simulink library "IOBlock_Library_TTC580"  (R2021a)
settings: Solver=ode45  StartTime=0.0  StopTime=10.0  RelTol=1e-3
PreLoadFcn:
  | addpath(genpath(fileparts(which('IOBlock_Library_TTC580'))));
  | %addpath(genpath(fileparts(which('IOBlock_Library_TTC580.mdl'))))
  | try
  | addpath(genpath([fileparts(which('IOBlock_Library_TTC580')),'\..\DBC_Importer']));
  | addpath(genpath([fileparts(which('IOBlock_Library_TTC580')),'\..\EEPROM_Importer']));
  | addpath(genpath([fileparts(which('IOBlock_Library_TTC580')),'\..\UserDoc']));
  | catch
  | warning('IOBlock_Library_TTC580: add path to DBC_Importer and EEPROM_Importer manually');
  | end
  | try
  | if exist('..\CustomPackage\scripts\OpenAllPackages.m','file')
  |      run('..\CustomPackage\scripts\OpenAllPackages.m'); %always available, ggf. empty
  | end
  | catch
  | warning('A problem occurred opening automatically the CustomPackage. Please open libraries manually');
  | end
  | try
  | set_param(0,'EditorSmartEditingHotParam','off');
  | catch
  | warning('Simlink preferences for ''Edit key parameter when adding new blocks'' needs to be unchecked manually');
  | end
undefined symbols (not defined in the file or in its folder): ADC_Absolute_10V, ADC_Absolute_32V, ADC_Absolute_5V, ADC_BoardTemp, ADC_ChannelInit, ADC_Current, ADC_Get, ADC_K15_, ADC_Ratiometric_10V, ADC_Ratiometric_5V, ADC_Resistive, ADC_SensorSupply, ADC_UBAT, bit_packing, bit_unpacking, CAN_ConfigMsg, compare2error, compare2FET_PROT_REENABLE, crc32_calc_intern, CRC32_EEPROM_Read, CRC32_EEPROM_Write, DIAG_EnterSafestate, DIAG_Status, DIAG_Status_internal, EEPROM_Mirror, EEPROM_Read, EEPROM_Read_OffsetIn, EEPROM_Read_Raw, EEPROM_Write, EEPROM_Write_OffsetIn, EEPROM_Write_Raw, EnterSafestate, FPU_Handler, Get_DI, Get_DI_VarThreshold, Get_K15_, Get_Pulse_Freq_Curr, Get_Pulse_Freq_Volt, Get_WakeUp, GetDateAndTime, IO_ADC_ResetProtection, IO_Blk_Lib_TTC500, IO_CAN_ReadMsg, IO_CAN_WriteMsg, IO_DI_Get, IO_DI_Init, IO_DI_Init_Var, IO_DO_GetCur, IO_DO_GetVoltage, IO_DO_Init, IO_DO_ResetProtection, IO_DO_Set, IO_Driver_GetSerialNumber, IO_Driver_GetVersionOfDriver, IO_Driver_GetVersionOfFPGA, IO_EEPROM_GetStatus, IO_EEPROM_Init, IO_EEPROM_Read_raw, IO_EEPROM_Write, IO_EEPROM_Write_OffsetIn ... (+73)
libraries: simulink x43
(part 5 of 18)

== system IOBlock_Library_TTC580/System  Blocks TTC580 IOlib ==
  DIAG_Status : Subsystem  LoadFcn=|  mask(DIAG_Status_Code){SampleTime=-1, ttlib=IO_Blk_Lib_TTC500, ttDescription=DIAG_Status, tt_iolib_version=0.16, FPGA_Major=16, FPGA_Minor=5, IODriver_Major=3, IODriver_Minor=1}
      | try
      | %specific upgrade to 0.15
      | if (0.15 > str2num(get_param(gcb,'tt_iolib_version'))) || (0.8 == str2num(get_param(gcb,'tt_iolib_version')))
      |    set_param(gcb,'IODriver_Minor','8'); 
      | end
      | %Upgrade Information - standard BEGIN
      | new_color = 'blue';
      | new_ver = '0.16';
      | act_ver = get_param(gcb,'tt_iolib_version');
      | if not(strcmp(act_ver,new_ver))
      |     disp(['Upgrade block: ',gcb,char(10),'       Version: ',act_ver,' -> ',new_ver]);
      |     %switch - case for specific upgrade information e.g. additional parameter required 
      |     %Change appearance and version information
      |     set_param(gcb,'ForegroundColor',new_color);
      |     set_param(gcb,'tt_iolib_version',new_ver);
      | end
      | %Upgrade Information - standard END
      | catch
      | %Standard catch section BEGIN 
      | disp(' ');
      | disp('------------------------------------------------------------');
      | disp('An error occurred in a callback of the TTC580-BlockLib.');
      | disp(['Please check the parameters in the mask of ',gcb]);
      | disp('If you do not encounter any violations, then please '); 
      | disp('copy the following lines and report this to support@ttcontrol.com ');
      | disp('<< begin of error message dump >>');
      | disp(['Version of TTC580-BlockLib: ', get_param(gcb,'tt_iolib_version')]);
      | disp(get_param(gcb,'ttDescription'));
      | disp(gcb);
      | x=lasterror;disp(x.message);
      | disp(get_param(gcb,'MaskValues'));
      | disp(version);
      | disp(computer);
      | disp('<< end of error message dump >>');
      | disp('------------------------------------------------------------');
      | disp(' ');
      | %Standard catch section END
      | end
      mask help: Status function for diagnostic state machine and watchdog states.
      mask init:
      | %
      settings: CopyFcn=%deleted
      mask Help: web([which('usermanual.html'),'#',lower(get_param(gcb,'ttDescription'))])
      mask Callback FPGA_Major: %
      mask Callback FPGA_Minor: %
      mask Callback IODriver_Major: %
      mask Callback IODriver_Minor: %
  EnterSafestate : Subsystem  mask(EnterSafestate_Code){SampleTime=-1, ttlib=IO_Blk_Lib_TTC500, ttDescription=EnterSafestate, tt_iolib_version=0.8}
      mask help: Allows an application driven safe state.
      mask init:
      | %
      settings: CopyFcn=%deleted
      mask Help: web([which('usermanual.html'),'#',lower(get_param(gcb,'ttDescription'))])
  FPU_Handler : Subsystem  LoadFcn=|  mask(FPU_Handler_Code){SampleTime=-1, ttlib=IO_Blk_Lib_TTC500, ttDescription=FPU_Handler, tt_iolib_version=0.25, division_by_zero=on, input_denormal=off, invalid_operation=on, overflow=on, underflow=off}
      | try
      | %
      | %Upgrade Information - standard BEGIN
      | new_color = 'blue';
      | new_ver = '0.25';
      | act_ver = get_param(gcb,'tt_iolib_version');
      | if not(strcmp(act_ver,new_ver))
      |     disp(['Upgrade block: ',gcb,char(10),'       Version: ',act_ver,' to ',new_ver]);
      |     %switch - case for specific upgrade information e.g. additional parameter required 
      |     %Change appearance and version information
      |     set_param(gcb,'ForegroundColor',new_color);
      |     set_param(gcb,'tt_iolib_version',new_ver);
      | end
      | %Upgrade Information - standard END
      | catch
      | %Standard catch section BEGIN
      | errordlg('An error occurred in a callback of the TTC580-BlockLib. Please open the Diagnostic Viewer for further details');
      | disp(' ');
      | disp('------------------------------------------------------------');
      | disp('An error occurred in a callback of the TTC580-BlockLib.');
      | disp(['Please check the parameters in the mask of ',gcb]);
      | disp('If you do not encounter any violations, then please '); 
      | disp('copy the following lines and report this to support@ttcontrol.com ');
      | disp('<< begin of error message dump >>');
      | disp(['Version of TTC580-BlockLib: ', get_param(gcb,'tt_iolib_version')]);
      | disp(get_param(gcb,'ttDescription'));
      | disp(gcb);
      | x=lasterror;disp(x.message);
      | disp(get_param(gcb,'MaskValues'));
      | disp(version);
      | disp(computer);
      | disp('<< end of error message dump >>');
      | disp('------------------------------------------------------------');
      | disp(' ');
      | %Standard catch section END
      | end
      mask help: Function for FPU exception handler.
      mask init:
      | %
      settings: CopyFcn=%deleted
      mask Help: web([which('usermanual.html'),'#',lower(get_param(gcb,'ttDescription'))])
      mask Callback division_by_zero: %
      mask Callback input_denormal: %
      mask Callback invalid_operation: %
      mask Callback overflow: %
      mask Callback underflow: %
  GetDateAndTime : Subsystem  LoadFcn=|  mask(GetDateAndTime_Code){SampleTime=-1, ttlib=IO_Blk_Lib_TTC500, ttDescription=GetDateAndTime, tt_iolib_version=0.18}
      | try
      | %
      | %Upgrade Information - standard BEGIN
      | new_color = 'blue';
      | new_ver = '0.18';
      | act_ver = get_param(gcb,'tt_iolib_version');
      | if not(strcmp(act_ver,new_ver))
      |     disp(['Upgrade block: ',gcb,char(10),'       Version: ',act_ver,' -> ',new_ver]);
      |     %switch - case for specific upgrade information e.g. additional parameter required 
      |     %Change appearance and version information
      |     set_param(gcb,'ForegroundColor',new_color);
      |     set_param(gcb,'tt_iolib_version',new_ver);
      | end
      | %Upgrade Information - standard END
      | catch
      | %Standard catch section BEGIN 
      | disp(' ');
      | disp('------------------------------------------------------------');
      | disp('An error occurred in a callback of the TTC580-BlockLib.');
      | disp(['Please check the parameters in the mask of ',gcb]);
      | disp('If you do not encounter any violations, then please '); 
      | disp('copy the following lines and report this to support@ttcontrol.com ');
      | disp('<< begin of error message dump >>');
      | disp(['Version of TTC580-BlockLib: ', get_param(gcb,'tt_iolib_version')]);
      | disp(get_param(gcb,'ttDescription'));
      | disp(gcb);
      | x=lasterror;disp(x.message);
      | disp(get_param(gcb,'MaskValues'));
      | disp(version);
      | disp(computer);
      | disp('<< end of error message dump >>');
      | disp('------------------------------------------------------------');
      | disp(' ');
      | %Standard catch section END
      | end
      mask help: Returns the date and time of the real time clock.
      mask init:
      | %
      settings: CopyFcn=%deleted
      mask Help: web([which('usermanual.html'),'#',lower(get_param(gcb,'ttDescription'))])
  IO_Driver_GetSerialNumber : Subsystem  LoadFcn=|  mask(IO_Driver_GetSerialNumber_Code){SampleTime=-1, ttlib=IO_Blk_Lib_TTC500, ttDescription=IO_Driver_GetSerialNumber, tt_iolib_version=0.24}
      | try
      | %
      | %Upgrade Information - standard BEGIN
      | new_color = 'blue';
      | new_ver = '0.24';
      | act_ver = get_param(gcb,'tt_iolib_version');
      | if not(strcmp(act_ver,new_ver))
      |     disp(['Upgrade block: ',gcb,char(10),'       Version: ',act_ver,' -> ',new_ver]);
      |     %switch - case for specific upgrade information e.g. additional parameter required 
      |     %Change appearance and version information
      |     set_param(gcb,'ForegroundColor',new_color);
      |     set_param(gcb,'tt_iolib_version',new_ver);
      | end
      | %Upgrade Information - standard END
      | catch
      | %Standard catch section BEGIN 
      | disp(' ');
      | disp('------------------------------------------------------------');
      | disp('An error occurred in a callback of the TTC580-BlockLib.');
      | disp(['Please check the parameters in the mask of ',gcb]);
      | disp('If you do not encounter any violations, then please '); 
      | disp('copy the following lines and report this to support@ttcontrol.com ');
      | disp('<< begin of error message dump >>');
      | disp(['Version of TTC580-BlockLib: ', get_param(gcb,'tt_iolib_version')]);
      | disp(get_param(gcb,'ttDescription'));
      | disp(gcb);
      | x=lasterror;disp(x.message);
      | disp(get_param(gcb,'MaskValues'));
      | disp(version);
      | disp(computer);
      | disp('<< end of error message dump >>');
      | disp('------------------------------------------------------------');
      | disp(' ');
      | %Standard catch section END
      | end
      mask help: Returns the ECU’s serial number.
      mask init:
      | %
      settings: CopyFcn=%deleted
      mask Help: web([which('usermanual.html'),'#',lower(get_param(gcb,'ttDescription'))])
  MainDlg : Subsystem  LoadFcn=|  mask(MainDlg_CCP_J1939__Code){SampleTime=-1, ttlib=IO_Blk_Lib_TTC500, ttDescription=MainDlg, tt_iolib_version=0.25, baudrate_CAN0=500, tseg1_CAN0=6, tseg2_CAN0=2, sjw_CAN0=1, brp_CAN0=1, baudrate_CAN1=500, tseg1_CAN1=6, tseg2_CAN1=2, sjw_CAN1=1, brp_CAN1=1, baudrate_CAN2=500, tseg1_CAN2=6, tseg2_CAN2=2, sjw_CAN2=1, brp_CAN2=1, baudrate_CAN3=500, baudrate_CAN4=500, baudrate_CAN5=500, baudrate_CAN6=500, tseg1=6, tseg2=2, sjw=1, Duration_ms=10, glitch_filter_time=180, watchdog_window_size=SAFETY_CONF_WINDOW_SIZE_100_PERCENT, watchdog_reset_behavior=SAFETY_CONF_RESETS_DISABLED, brp=0, Enable_sending_DM1_of_J1939=off, DM1_Channel=IO_CAN_CHANNEL_0, J1939SorceAddress=0, DM2_Basis_Address=63488, Show_version_information=off, Major_Number=0, Minor_Number=1, Revison_Number=1, Node_Number=1, Enable_Reset_by_TTCDownloader=on, bFlashOverEthernet=off, Enable_CCP=off, CRO_ID=hex2dec('101'), DTO_ID=hex2dec('102'), CCP_Station_Addr_raw=1, CCP_Station_ID=ECU00001, CPP_channel=IO_CAN_CHANNEL_0, CPP_id_format=IO_CAN_STD_FRAME, bEnable_DAQ0=off, bEnable_DAQ1_2=off, ODT_total=10, bEnable_ErrorCBAction=off, bDIAG_ERR_DISABLE_SSW0=off, bDIAG_ERR_DISABLE_SSW1=off, bDIAG_ERR_DISABLE_SSW2=off}
      | try
      | %
      | %Upgrade Information - standard BEGIN
      | new_color = 'blue';
      | new_ver = '0.25';
      | act_ver = get_param(gcb,'tt_iolib_version');
      | if not(strcmp(act_ver,new_ver))
      |     disp(['Upgrade block: ',gcb,char(10),'       Version: ',act_ver,' to ',new_ver]);
      |     %switch - case for specific upgrade information e.g. additional parameter required 
      |     %Change appearance and version information
      |     set_param(gcb,'ForegroundColor',new_color);
      |     set_param(gcb,'tt_iolib_version',new_ver);
      | end
      | %Upgrade Information - standard END
      | catch
      | %Standard catch section BEGIN
      | errordlg('An error occurred in a callback of the TTC580-BlockLib. Please open the Diagnostic Viewer for further details');
      | disp(' ');
      | disp('------------------------------------------------------------');
      | disp('An error occurred in a callback of the TTC580-BlockLib.');
      | disp(['Please check the parameters in the mask of ',gcb]);
      | disp('If you do not encounter any violations, then please '); 
      | disp('copy the following lines and report this to support@ttcontrol.com ');
      | disp('<< begin of error message dump >>');
      | disp(['Version of TTC580-BlockLib: ', get_param(gcb,'tt_iolib_version')]);
      | disp(get_param(gcb,'ttDescription'));
      | disp(gcb);
      | x=lasterror;disp(x.message);
      | disp(get_param(gcb,'MaskValues'));
      | disp(version);
      | disp(computer);
      | disp('<< end of error message dump >>');
      | disp('------------------------------------------------------------');
      | disp(' ');
      | %Standard catch section END
      | end
      mask prompts: tseg1_CAN0 "tseg1 for CAN0"; tseg2_CAN0 "tseg2 for CAN0"; sjw_CAN0 "sjw for CAN0"; brp_CAN0 "brp for CAN0"; tseg1_CAN1 "tseg1 for CAN1"; tseg2_CAN1 "tseg2 for CAN1"; sjw_CAN1 "sjw for CAN1"; brp_CAN1 "brp for CAN1"; tseg1_CAN2 "tseg1 for CAN2"; tseg2_CAN2 "tseg2 for CAN2"; sjw_CAN2 "sjw for CAN2"; brp_CAN2 "brp for CAN2"; Enable_sending_DM1_of_J1939 "Enable DMx services (J1939)"; DM1_Channel "J1939 channel"; DM2_Basis_Address "Basis Address DM2 [0..63488]"; Show_version_information "Show additional information"; Major_Number "Major Number:"; Minor_Number "Minor Number:"; Revison_Number "Revision Number:"; Node_Number "Node Number:"; Enable_Reset_by_TTCDownloader "Reset by TTC-Downloader"; bFlashOverEthernet "Enable ethernet download requests"; Enable_CCP "Enable CCP"; CRO_ID "CRO ID"; DTO_ID "DTO ID"; CCP_Station_Addr_raw "CCP Station Address"; CCP_Station_ID "CCP Station ID"; CPP_channel "CPP channel"; CPP_id_format "CRO DTO Id format"; bEnable_DAQ0 "Enable DAQ sync"; bEnable_DAQ1_2 "Enable DAQ alternate"; ODT_total "Total ODTs for DAQ lists"; bEnable_ErrorCBAction "Enable dedicated actions for error callback"; bDIAG_ERR_DISABLE_SSW0 "Shut-off group 0"; bDIAG_ERR_DISABLE_SSW1 "Shut-off group 1"; bDIAG_ERR_DISABLE_SSW2 "Shut-off group 2"
      mask help: Block representing main environment-settings of the applications to be run on a TTC580.
      mask init:
      | try
      | %Check if the selected channel is set to 250kBit/s
      | if strcmp(get_param(gcb,'Enable_sending_DM1_of_J1939'),'on')
      |  sChannel = get_param(gcb, 'DM1_Channel');   
      |  cChannelNumber = regexp(sChannel,'(\d)*','match');  %extract numbers
      |  sChannelNumber =  cChannelNumber{end}; %take last number
      |  if ~strcmp(get_param(gcb,['baudrate_CAN',sChannelNumber]),'250')
      |    disp('TTC580-Lib Warning for MainDlg Block: ');
      |    disp(['Setting for baudrate_CAN',sChannelNumber,' is not 250kBit/s as defined in J1939 standard']);
      |    disp('!!!'); 
      | end
      | end
      | if (Duration_ms > 50) || (Duration_ms < 1)
      |     disp('Duration_ms is chosen out of bounds [1..50] !!!');
      | end
      | %swap the Station Address because of Intel format representation due to CCP specification
      | CCP_Station_Addr_raw_loc = str2num(get_param(gcb,'CCP_Station_Addr_raw'));
      | CCP_Station_Addr = swapbytes(uint16(CCP_Station_Addr_raw_loc));%because of big-endian format on the TMS570
      | %%CT>
      | TAG_loc = get_param(gcb,'Tag');
      | if ~isempty(TAG_loc),[~,y]=regexp(TAG_loc,'(^[a-zA-Z0-9_]*)');
      |     if isempty(y) || y~=builtin('length',(TAG_loc)) %don't use length() alone!
      |         error(['The Tag: ',TAG_loc,' needs to start with a letter and may only contain the characters 0-9,a-Z,_ .']);
      | end,end
      | x=find_system(gcbh,'FollowLinks','on','LookUnderMasks','on','BlockType','S-Function');
      | for i=1:builtin('length',(x)) %don't use length() alone!
      |     set_param(x(i),'Tag',TAG_loc);
      | end
      | %<CT%
      | 
      | catch
      | %Standard catch section BEGIN
      | errordlg('An error occurred in a callback of the TTC580-BlockLib. Please open the Diagnostic Viewer for further details');
      | disp(' ');
      | disp('------------------------------------------------------------');
      | disp('An error occurred in a callback of the TTC580-BlockLib.');
      | disp(['Please check the parameters in the mask of ',gcb]);
      | disp('If you do not encounter any violations, then please '); 
      | disp('copy the following lines and report this to support@ttcontrol.com ');
      | disp('<< begin of error message dump >>');
      | disp(['Version of TTC580-BlockLib: ', get_param(gcb,'tt_iolib_version')]);
      | disp(get_param(gcb,'ttDescription'));
      | disp(gcb);
      | x=lasterror;disp(x.message);
      | disp(get_param(gcb,'MaskValues'));
      | disp(version);
      | disp(computer);
      | disp('<< end of error message dump >>');
      | disp('------------------------------------------------------------');
      | disp(' ');
      | %Standard catch section END
      | end
      settings: CopyFcn=%deleted
      mask Help: web([which('usermanual.html'),'#',lower(get_param(gcb,'ttDescription'))])
      mask TypeOptions baudrate_CAN0: 50 | 100 | 125 | 250 | 500 | 1000 | IO_CAN_BIT_USER
      mask Callback baudrate_CAN0:
      | try
      | s_ParameterDecision = 'baudrate_CAN0'; %Deside on this parameter
      | c_ValuesDecision={'50','100','125','250','500','1000'}; %Positive DescitionValues
      | s_ParameterInvisible = {'tseg1_CAN0','tseg2_CAN0','brp_CAN0'}; %Make this invisible
      | %trim
      | if ischar(s_ParameterInvisible)%if secttion for compatibility reasons of template
      |     cs_ParameterInvisible = {s_ParameterInvisible};
      | else
      |     cs_ParameterInvisible = s_ParameterInvisible;
      | end
      | s_ParameterDecision = strtrim(s_ParameterDecision);
      | c_ValuesDecision = strtrim(c_ValuesDecision);
      | for j=1:length(cs_ParameterInvisible)
      |   s_ParameterInvisible = strtrim(cs_ParameterInvisible{j});
      |   c_MaskVisibilities=get_param(gcb,'MaskVisibilities');
      |   %check consistency
      |   idx=strmatch(s_ParameterInvisible,get_param(gcb,'MaskNames'),'exact');
      |   c_MaskVisibilities{idx}='on'; %default
      |     for i = 1: length(c_ValuesDecision)
      |         if ~isempty(strmatch(get_param(gcb, s_ParameterDecision), c_ValuesDecision{i},'exact'))
      |            c_MaskVisibilities{idx}='off';
      |         end
      |     end
      |   set_param(gcb,'MaskVisibilities',c_MaskVisibilities);
      | end
      | catch
      | %Standard catch section BEGIN
      | errordlg('An error occurred in a callback of the TTC580-BlockLib. Please open the Diagnostic Viewer for further details');
      | disp(' ');
      | disp('------------------------------------------------------------');
      | disp('An error occurred in a callback of the TTC580-BlockLib.');
      | disp(['Please check the parameters in the mask of ',gcb]);
      | disp('If you do not encounter any violations, then please ');
      | disp('copy the following lines and report this to support@ttcontrol.com ');
      | disp('<< begin of error message dump >>');
      | disp(['Version of TTC580-BlockLib: ', get_param(gcb,'tt_iolib_version')]);
      | disp(get_param(gcb,'ttDescription'));
      | disp(gcb);
      | x=lasterror;disp(x.message);
      | disp(get_param(gcb,'MaskValues'));
      | disp(version);
      | disp(computer);
      | disp('<< end of error message dump >>');
      | disp('------------------------------------------------------------');
      | disp(' ');
      | %Standard catch section END
      | end
      mask TypeOptions tseg1_CAN0: 3 | 4 | 5 | 6 | 7 | 8 | 9 | 10 | 11 | 12 | 13 | 14 | 15 | 16
      mask Callback tseg1_CAN0: %
      mask TypeOptions tseg2_CAN0: 2 | 3 | 4 | 5 | 6 | 7 | 8
      mask Callback tseg2_CAN0: %
      mask TypeOptions sjw_CAN0: 1 | 2 | 3 | 4
      mask Callback sjw_CAN0: %
      mask TypeOptions brp_CAN0: 1 | 2 | 3 | 4 | 5 | 6 | 7 | 8 | 9 | 10 | 11 | 12 | 13 | 14 | 15 | 16 | 17 | 18 | 19 | 20 | 21 | 22 | 23 | 24 | 25 | 26 | 27 | 28 | 29 | 30 | 31 | 32 | 33 | 34 | 35 | 36 | 37 | 38 | 39 | 40 | 41 | 42 | 43 | 44 | 45 | 46 | 47 | 48 | 49 | 50 | 51 | 52 | 53 | 54 | 55 | 56 | 57 | 58 | 59 | 60 | 61 | 62 | 63 | 64
      mask Callback brp_CAN0: %
      mask TypeOptions baudrate_CAN1: 50 | 100 | 125 | 250 | 500 | 1000 | IO_CAN_BIT_USER
      mask Callback baudrate_CAN1:
      | try
      | s_ParameterDecision = 'baudrate_CAN1'; %Deside on this parameter
      | c_ValuesDecision={'50','100','125','250','500','1000'}; %Positive DescitionValues
      | s_ParameterInvisible = {'tseg1_CAN1','tseg2_CAN1','brp_CAN1'}; %Make this invisible
      | %trim
      | if ischar(s_ParameterInvisible)%if secttion for compatibility reasons of template
      |     cs_ParameterInvisible = {s_ParameterInvisible};
      | else
      |     cs_ParameterInvisible = s_ParameterInvisible;
      | end
      | s_ParameterDecision = strtrim(s_ParameterDecision);
      | c_ValuesDecision = strtrim(c_ValuesDecision);
      | for j=1:length(cs_ParameterInvisible)
      |   s_ParameterInvisible = strtrim(cs_ParameterInvisible{j});
      |   c_MaskVisibilities=get_param(gcb,'MaskVisibilities');
      |   %check consistency
      |   idx=strmatch(s_ParameterInvisible,get_param(gcb,'MaskNames'),'exact');
      |   c_MaskVisibilities{idx}='on'; %default
      |     for i = 1: length(c_ValuesDecision)
      |         if ~isempty(strmatch(get_param(gcb, s_ParameterDecision), c_ValuesDecision{i},'exact'))
      |            c_MaskVisibilities{idx}='off';
      |         end
      |     end
      |   set_param(gcb,'MaskVisibilities',c_MaskVisibilities);
      | end
      | catch
      | %Standard catch section BEGIN
      | errordlg('An error occurred in a callback of the TTC580-BlockLib. Please open the Diagnostic Viewer for further details');
      | disp(' ');
      | disp('------------------------------------------------------------');
      | disp('An error occurred in a callback of the TTC580-BlockLib.');
      | disp(['Please check the parameters in the mask of ',gcb]);
      | disp('If you do not encounter any violations, then please ');
      | disp('copy the following lines and report this to support@ttcontrol.com ');
      | disp('<< begin of error message dump >>');
      | disp(['Version of TTC580-BlockLib: ', get_param(gcb,'tt_iolib_version')]);
      | disp(get_param(gcb,'ttDescription'));
      | disp(gcb);
      | x=lasterror;disp(x.message);
      | disp(get_param(gcb,'MaskValues'));
      | disp(version);
      | disp(computer);
      | disp('<< end of error message dump >>');
      | disp('------------------------------------------------------------');
      | disp(' ');
      | %Standard catch section END
      | end
      mask TypeOptions tseg1_CAN1: 3 | 4 | 5 | 6 | 7 | 8 | 9 | 10 | 11 | 12 | 13 | 14 | 15 | 16
      mask Callback tseg1_CAN1: %
      mask TypeOptions tseg2_CAN1: 2 | 3 | 4 | 5 | 6 | 7 | 8
      mask Callback tseg2_CAN1: %
      mask TypeOptions sjw_CAN1: 1 | 2 | 3 | 4
      mask Callback sjw_CAN1: %
      mask TypeOptions brp_CAN1: 1 | 2 | 3 | 4 | 5 | 6 | 7 | 8 | 9 | 10 | 11 | 12 | 13 | 14 | 15 | 16 | 17 | 18 | 19 | 20 | 21 | 22 | 23 | 24 | 25 | 26 | 27 | 28 | 29 | 30 | 31 | 32 | 33 | 34 | 35 | 36 | 37 | 38 | 39 | 40 | 41 | 42 | 43 | 44 | 45 | 46 | 47 | 48 | 49 | 50 | 51 | 52 | 53 | 54 | 55 | 56 | 57 | 58 | 59 | 60 | 61 | 62 | 63 | 64
      mask Callback brp_CAN1: %
      mask TypeOptions baudrate_CAN2: 50 | 100 | 125 | 250 | 500 | 1000 | IO_CAN_BIT_USER
      mask Callback baudrate_CAN2:
      | try
      | s_ParameterDecision = 'baudrate_CAN2'; %Deside on this parameter
      | c_ValuesDecision={'50','100','125','250','500','1000'}; %Positive DescitionValues
      | s_ParameterInvisible = {'tseg1_CAN2','tseg2_CAN2','brp_CAN2'}; %Make this invisible
      | %trim
      | if ischar(s_ParameterInvisible)%if secttion for compatibility reasons of template
      |     cs_ParameterInvisible = {s_ParameterInvisible};
      | else
      |     cs_ParameterInvisible = s_ParameterInvisible;
      | end
      | s_ParameterDecision = strtrim(s_ParameterDecision);
      | c_ValuesDecision = strtrim(c_ValuesDecision);
      | for j=1:length(cs_ParameterInvisible)
      |   s_ParameterInvisible = strtrim(cs_ParameterInvisible{j});
      |   c_MaskVisibilities=get_param(gcb,'MaskVisibilities');
      |   %check consistency
      |   idx=strmatch(s_ParameterInvisible,get_param(gcb,'MaskNames'),'exact');
      |   c_MaskVisibilities{idx}='on'; %default
      |     for i = 1: length(c_ValuesDecision)
      |         if ~isempty(strmatch(get_param(gcb, s_ParameterDecision), c_ValuesDecision{i},'exact'))
      |            c_MaskVisibilities{idx}='off';
      |         end
      |     end
      |   set_param(gcb,'MaskVisibilities',c_MaskVisibilities);
      | end
      | catch
      | %Standard catch section BEGIN
      | errordlg('An error occurred in a callback of the TTC580-BlockLib. Please open the Diagnostic Viewer for further details');
      | disp(' ');
      | disp('------------------------------------------------------------');
      | disp('An error occurred in a callback of the TTC580-BlockLib.');
      | disp(['Please check the parameters in the mask of ',gcb]);
      | disp('If you do not encounter any violations, then please ');
      | disp('copy the following lines and report this to support@ttcontrol.com ');
      | disp('<< begin of error message dump >>');
      | disp(['Version of TTC580-BlockLib: ', get_param(gcb,'tt_iolib_version')]);
      | disp(get_param(gcb,'ttDescription'));
      | disp(gcb);
      | x=lasterror;disp(x.message);
      | disp(get_param(gcb,'MaskValues'));
      | disp(version);
      | disp(computer);
      | disp('<< end of error message dump >>');
      | disp('------------------------------------------------------------');
      | disp(' ');
      | %Standard catch section END
      | end
      mask TypeOptions tseg1_CAN2: 3 | 4 | 5 | 6 | 7 | 8 | 9 | 10 | 11 | 12 | 13 | 14 | 15 | 16
      mask Callback tseg1_CAN2: %
      mask TypeOptions tseg2_CAN2: 2 | 3 | 4 | 5 | 6 | 7 | 8
      mask Callback tseg2_CAN2: %
      mask TypeOptions sjw_CAN2: 1 | 2 | 3 | 4
      mask Callback sjw_CAN2: %
      mask TypeOptions brp_CAN2: 1 | 2 | 3 | 4 | 5 | 6 | 7 | 8 | 9 | 10 | 11 | 12 | 13 | 14 | 15 | 16 | 17 | 18 | 19 | 20 | 21 | 22 | 23 | 24 | 25 | 26 | 27 | 28 | 29 | 30 | 31 | 32 | 33 | 34 | 35 | 36 | 37 | 38 | 39 | 40 | 41 | 42 | 43 | 44 | 45 | 46 | 47 | 48 | 49 | 50 | 51 | 52 | 53 | 54 | 55 | 56 | 57 | 58 | 59 | 60 | 61 | 62 | 63 | 64
      mask Callback brp_CAN2: %
      mask TypeOptions baudrate_CAN3: 50 | 100 | 125 | 250 | 500 | 1000
      mask Callback baudrate_CAN3: %
      mask TypeOptions baudrate_CAN4: 50 | 100 | 125 | 250 | 500 | 1000
      mask Callback baudrate_CAN4: %
      mask TypeOptions baudrate_CAN5: 50 | 100 | 125 | 250 | 500 | 1000
      mask Callback baudrate_CAN5: %
      mask TypeOptions baudrate_CAN6: 50 | 100 | 125 | 250 | 500 | 1000
      mask Callback baudrate_CAN6: %
      mask TypeOptions tseg1: 3 | 4 | 5 | 6 | 7 | 8 | 9 | 10 | 11 | 12 | 13 | 14 | 15 | 16
      mask Callback tseg1: %
      mask TypeOptions tseg2: 2 | 3 | 4 | 5 | 6 | 7 | 8
      mask Callback tseg2: %
      mask TypeOptions sjw: 1 | 2 | 3 | 4
      mask Callback sjw: %
      mask Callback Duration_ms: %
      mask Callback glitch_filter_time: %
      mask TypeOptions watchdog_window_size: SAFETY_CONF_WINDOW_SIZE_100_PERCENT | SAFETY_CONF_WINDOW_SIZE_50_PERCENT | SAFETY_CONF_WINDOW_SIZE_25_PERCENT | SAFETY_CONF_WINDOW_SIZE_12_5_PERCENT | SAFETY_CONF_WINDOW_SIZE_6_25_PERCENT | SAFETY_CONF_WINDOW_SIZE_3_125_PERCENT
      mask Callback watchdog_window_size: %
      mask Callback watchdog_reset_behavior: %
      mask Callback brp: %
      mask Callback Enable_sending_DM1_of_J1939:
      | try
      | s_ParameterDecision = 'Enable_sending_DM1_of_J1939'; %Deside on this parameter
      | c_ValuesDecision={'off'}; %Positive DescitionValues
      | s_ParameterInvisible = 'DM1_Channel'; %Make this invisible
      | %trim
      | if ischar(s_ParameterInvisible)%if secttion for compatibility reasons of template
      |     cs_ParameterInvisible = {s_ParameterInvisible};
      | else
      |     cs_ParameterInvisible = s_ParameterInvisible;
      | end
      | s_ParameterDecision = strtrim(s_ParameterDecision);
      | c_ValuesDecision = strtrim(c_ValuesDecision);
      | for j=1:length(cs_ParameterInvisible)
      |   s_ParameterInvisible = strtrim(cs_ParameterInvisible{j});
      |   c_MaskVisibilities=get_param(gcb,'MaskVisibilities');
      |   %check consistency
      |   idx=strmatch(s_ParameterInvisible,get_param(gcb,'MaskNames'),'exact');
      |   c_MaskVisibilities{idx}='on'; %default
      |     for i = 1: length(c_ValuesDecision)
      |         if ~isempty(strmatch(get_param(gcb, s_ParameterDecision), c_ValuesDecision{i},'exact'))
      |            c_MaskVisibilities{idx}='off';
      |         end
      |     end
      |   set_param(gcb,'MaskVisibilities',c_MaskVisibilities);
      | end
      | s_ParameterDecision = 'Enable_sending_DM1_of_J1939'; %Deside on this parameter
      | c_ValuesDecision={'off'}; %Positive DescitionValues
      | s_ParameterInvisible = 'J1939SorceAddress'; %Make this invisible
      | %trim
      | if ischar(s_ParameterInvisible)%if secttion for compatibility reasons of template
      |     cs_ParameterInvisible = {s_ParameterInvisible};
      | else
      |     cs_ParameterInvisible = s_ParameterInvisible;
      | end
      | s_ParameterDecision = strtrim(s_ParameterDecision);
      | c_ValuesDecision = strtrim(c_ValuesDecision);
      | for j=1:length(cs_ParameterInvisible)
      |   s_ParameterInvisible = strtrim(cs_ParameterInvisible{j});
      |   c_MaskVisibilities=get_param(gcb,'MaskVisibilities');
      |   %check consistency
      |   idx=strmatch(s_ParameterInvisible,get_param(gcb,'MaskNames'),'exact');
      |   c_MaskVisibilities{idx}='on'; %default
      |     for i = 1: length(c_ValuesDecision)
      |         if ~isempty(strmatch(get_param(gcb, s_ParameterDecision), c_ValuesDecision{i},'exact'))
      |            c_MaskVisibilities{idx}='off';
      |         end
      |     end
      |   set_param(gcb,'MaskVisibilities',c_MaskVisibilities);
      | end
      | s_ParameterDecision = 'Enable_sending_DM1_of_J1939'; %Deside on this parameter
      | c_ValuesDecision={'off'}; %Positive DescitionValues
      | s_ParameterInvisible = 'DM2_Basis_Address'; %Make this invisible
      | %trim
      | if ischar(s_ParameterInvisible)%if secttion for compatibility reasons of template
      |     cs_ParameterInvisible = {s_ParameterInvisible};
      | else
      |     cs_ParameterInvisible = s_ParameterInvisible;
      | end
      | s_ParameterDecision = strtrim(s_ParameterDecision);
      | c_ValuesDecision = strtrim(c_ValuesDecision);
      | for j=1:length(cs_ParameterInvisible)
      |   s_ParameterInvisible = strtrim(cs_ParameterInvisible{j});
      |   c_MaskVisibilities=get_param(gcb,'MaskVisibilities');
      |   %check consistency
      |   idx=strmatch(s_ParameterInvisible,get_param(gcb,'MaskNames'),'exact');
      |   c_MaskVisibilities{idx}='on'; %default
      |     for i = 1: length(c_ValuesDecision)
      |         if ~isempty(strmatch(get_param(gcb, s_ParameterDecision), c_ValuesDecision{i},'exact'))
      |            c_MaskVisibilities{idx}='off';
      |         end
      |     end
      |   set_param(gcb,'MaskVisibilities',c_MaskVisibilities);
      | end
      | catch
      | %Standard catch section BEGIN
      | errordlg('An error occurred in a callback of the TTC580-BlockLib. Please open the Diagnostic Viewer for further details');
      | disp(' ');
      | disp('------------------------------------------------------------');
      | disp('An error occurred in a callback of the TTC580-BlockLib.');
      | disp(['Please check the parameters in the mask of ',gcb]);
      | disp('If you do not encounter any violations, then please ');
      | disp('copy the following lines and report this to support@ttcontrol.com ');
      | disp('<< begin of error message dump >>');
      | disp(['Version of TTC580-BlockLib: ', get_param(gcb,'tt_iolib_version')]);
      | disp(get_param(gcb,'ttDescription'));
      | disp(gcb);
      | x=lasterror;disp(x.message);
      | disp(get_param(gcb,'MaskValues'));
      | disp(version);
      | disp(computer);
      | disp('<< end of error message dump >>');
      | disp('------------------------------------------------------------');
      | disp(' ');
      | %Standard catch section END
      | end
      mask TypeOptions DM1_Channel: IO_CAN_CHANNEL_0  | IO_CAN_CHANNEL_1 | IO_CAN_CHANNEL_2 | IO_CAN_CHANNEL_3 | IO_CAN_CHANNEL_4 | IO_CAN_CHANNEL_5 | IO_CAN_CHANNEL_6
      mask Callback DM1_Channel: %
      mask Callback J1939SorceAddress: %
      mask Callback DM2_Basis_Address:
      | try
      | sParam = 'DM2_Basis_Address';
      | vBounds = [0,63488];
      | iValue = str2num(get_param(gcb,sParam));
      | if (iValue > vBounds(2))
      |     disp(['Value of ',sParam,' is chosen out of bounds [',num2str(vBounds(1)),'..',num2str(vBounds(2)),'] -> set to maximum possible !!!']);
      |     iValue = vBounds(2); %set to maximum
      |     set_param(gcb,sParam,num2str(iValue));
      | elseif (iValue < vBounds(1))
      |     disp(['Value of ',sParam,' is chosen out of bounds [',num2str(vBounds(1)),'..',num2str(vBounds(2)),'] -> set to minimum possible !!!']);
      |     iValue = vBounds(1); %set to minimum
      |     set_param(gcb,sParam,num2str(iValue));
      | end
      | catch
      | %Standard catch section BEGIN
      | errordlg('An error occurred in a callback of the TTC580-BlockLib. Please open the Diagnostic Viewer for further details');
      | disp(' ');
      | disp('------------------------------------------------------------');
      | disp('An error occurred in a callback of the TTC580-BlockLib.');
      | disp(['Please check the parameters in the mask of ',gcb]);
      | disp('If you do not encounter any violations, then please ');
      | disp('copy the following lines and report this to support@ttcontrol.com ');
      | disp('<< begin of error message dump >>');
      | disp(['Version of TTC580-BlockLib: ', get_param(gcb,'tt_iolib_version')]);
      | disp(get_param(gcb,'ttDescription'));
      | disp(gcb);
      | x=lasterror;disp(x.message);
      | disp(get_param(gcb,'MaskValues'));
      | disp(version);
      | disp(computer);
      | disp('<< end of error message dump >>');
      | disp('------------------------------------------------------------');
      | disp(' ');
      | %Standard catch section END
      | end
      mask Callback Show_version_information:
      | try
      | s_ParameterDecision = 'Show_version_information'; %Deside on this parameter
      | c_ValuesDecision={'off'}; %Positive DescitionValues
      | s_ParameterInvisible = 'Major_Number'; %Make this invisible
      | %trim
      | if ischar(s_ParameterInvisible)%if secttion for compatibility reasons of template
      |     cs_ParameterInvisible = {s_ParameterInvisible};
      | else
      |     cs_ParameterInvisible = s_ParameterInvisible;
      | end
      | s_ParameterDecision = strtrim(s_ParameterDecision);
      | c_ValuesDecision = strtrim(c_ValuesDecision);
      | for j=1:length(cs_ParameterInvisible)
      |   s_ParameterInvisible = strtrim(cs_ParameterInvisible{j});
      |   c_MaskVisibilities=get_param(gcb,'MaskVisibilities');
      |   %check consistency
      |   idx=strmatch(s_ParameterInvisible,get_param(gcb,'MaskNames'),'exact');
      |   c_MaskVisibilities{idx}='on'; %default
      |     for i = 1: length(c_ValuesDecision)
      |         if ~isempty(strmatch(get_param(gcb, s_ParameterDecision), c_ValuesDecision{i},'exact'))
      |            c_MaskVisibilities{idx}='off';
      |         end
      |     end
      |   set_param(gcb,'MaskVisibilities',c_MaskVisibilities);
      | end
      | s_ParameterDecision = 'Show_version_information'; %Deside on this parameter
      | c_ValuesDecision={'off'}; %Positive DescitionValues
      | s_ParameterInvisible = 'Minor_Number'; %Make this invisible
      | %trim
      | if ischar(s_ParameterInvisible)%if secttion for compatibility reasons of template
      |     cs_ParameterInvisible = {s_ParameterInvisible};
      | else
      |     cs_ParameterInvisible = s_ParameterInvisible;
      | end
      | s_ParameterDecision = strtrim(s_ParameterDecision);
      | c_ValuesDecision = strtrim(c_ValuesDecision);
      | for j=1:length(cs_ParameterInvisible)
      |   s_ParameterInvisible = strtrim(cs_ParameterInvisible{j});
      |   c_MaskVisibilities=get_param(gcb,'MaskVisibilities');
      |   %check consistency
      |   idx=strmatch(s_ParameterInvisible,get_param(gcb,'MaskNames'),'exact');
      |   c_MaskVisibilities{idx}='on'; %default
      |     for i = 1: length(c_ValuesDecision)
      |         if ~isempty(strmatch(get_param(gcb, s_ParameterDecision), c_ValuesDecision{i},'exact'))
      |            c_MaskVisibilities{idx}='off';
      |         end
      |     end
      |   set_param(gcb,'MaskVisibilities',c_MaskVisibilities);
      | end
      | s_ParameterDecision = 'Show_version_information'; %Deside on this parameter
      | c_ValuesDecision={'off'}; %Positive DescitionValues
      | s_ParameterInvisible = 'Revison_Number'; %Make this invisible
      | %trim
      | if ischar(s_ParameterInvisible)%if secttion for compatibility reasons of template
      |     cs_ParameterInvisible = {s_ParameterInvisible};
      | else
      |     cs_ParameterInvisible = s_ParameterInvisible;
      | end
      | s_ParameterDecision = strtrim(s_ParameterDecision);
      | c_ValuesDecision = strtrim(c_ValuesDecision);
      | for j=1:length(cs_ParameterInvisible)
      |   s_ParameterInvisible = strtrim(cs_ParameterInvisible{j});
      |   c_MaskVisibilities=get_param(gcb,'MaskVisibilities');
      |   %check consistency
      |   idx=strmatch(s_ParameterInvisible,get_param(gcb,'MaskNames'),'exact');
      |   c_MaskVisibilities{idx}='on'; %default
      |     for i = 1: length(c_ValuesDecision)
      |         if ~isempty(strmatch(get_param(gcb, s_ParameterDecision), c_ValuesDecision{i},'exact'))
      |            c_MaskVisibilities{idx}='off';
      |         end
      |     end
      |   set_param(gcb,'MaskVisibilities',c_MaskVisibilities);
      | end
      | s_ParameterDecision = 'Show_version_information'; %Deside on this parameter
      | c_ValuesDecision={'off'}; %Positive DescitionValues
      | s_ParameterInvisible = 'Node_Number'; %Make this invisible
      | %trim
      | if ischar(s_ParameterInvisible)%if secttion for compatibility reasons of template
      |     cs_ParameterInvisible = {s_ParameterInvisible};
      | else
      |     cs_ParameterInvisible = s_ParameterInvisible;
      | end
      | s_ParameterDecision = strtrim(s_ParameterDecision);
      | c_ValuesDecision = strtrim(c_ValuesDecision);
      | for j=1:length(cs_ParameterInvisible)
      |   s_ParameterInvisible = strtrim(cs_ParameterInvisible{j});
      |   c_MaskVisibilities=get_param(gcb,'MaskVisibilities');
      |   %check consistency
      |   idx=strmatch(s_ParameterInvisible,get_param(gcb,'MaskNames'),'exact');
      |   c_MaskVisibilities{idx}='on'; %default
      |     for i = 1: length(c_ValuesDecision)
      |         if ~isempty(strmatch(get_param(gcb, s_ParameterDecision), c_ValuesDecision{i},'exact'))
      |            c_MaskVisibilities{idx}='off';
      |         end
      |     end
      |   set_param(gcb,'MaskVisibilities',c_MaskVisibilities);
      | end
      | catch
      | %Standard catch section BEGIN
      | errordlg('An error occurred in a callback of the TTC580-BlockLib. Please open the Diagnostic Viewer for further details');
      | disp(' ');
      | disp('------------------------------------------------------------');
      | disp('An error occurred in a callback of the TTC580-BlockLib.');
      | disp(['Please check the parameters in the mask of ',gcb]);
      | disp('If you do not encounter any violations, then please ');
      | disp('copy the following lines and report this to support@ttcontrol.com ');
      | disp('<< begin of error message dump >>');
      | disp(['Version of TTC580-BlockLib: ', get_param(gcb,'tt_iolib_version')]);
      | disp(get_param(gcb,'ttDescription'));
      | disp(gcb);
      | x=lasterror;disp(x.message);
      | disp(get_param(gcb,'MaskValues'));
      | disp(version);
      | disp(computer);
      | disp('<< end of error message dump >>');
      | disp('------------------------------------------------------------');
      | disp(' ');
      | %Standard catch section END
      | end
      mask Callback Major_Number: %
      mask Callback Minor_Number: %
      mask Callback Revison_Number: %
      mask Callback Node_Number: %
      mask Callback Enable_Reset_by_TTCDownloader:
      | try
      | s_ParameterDecision = 'Enable_Reset_by_TTCDownloader'; %Deside on this parameter
      | c_ValuesDecision={'on'}; %Positive DescitionValues
      | s_ParameterInvisible = 'bFlashOverEthernet'; %Make this invisible
      | %trim
      | if ischar(s_ParameterInvisible)%if secttion for compatibility reasons of template
      |     cs_ParameterInvisible = {s_ParameterInvisible};
      | else
      |     cs_ParameterInvisible = s_ParameterInvisible;
      | end
      | s_ParameterDecision = strtrim(s_ParameterDecision);
      | c_ValuesDecision = strtrim(c_ValuesDecision);
      | for j=1:length(cs_ParameterInvisible)
      |   s_ParameterInvisible = strtrim(cs_ParameterInvisible{j});
      |   c_MaskVisibilities=get_param(gcb,'MaskVisibilities');
      |   %check consistency
      |   idx=strmatch(s_ParameterInvisible,get_param(gcb,'MaskNames'),'exact');
      |   c_MaskVisibilities{idx}='on'; %default
      |     for i = 1: length(c_ValuesDecision)
      |         if ~isempty(strmatch(get_param(gcb, s_ParameterDecision), c_ValuesDecision{i},'exact'))
      |            c_MaskVisibilities{idx}='off';
      |         end
      |     end
      |   set_param(gcb,'MaskVisibilities',c_MaskVisibilities);
      | end
      | catch
      | %Standard catch section BEGIN
      | errordlg('An error occurred in a callback of the TTC580-BlockLib. Please open the Diagnostic Viewer for further details');
      | disp(' ');
      | disp('------------------------------------------------------------');
      | disp('An error occurred in a callback of the TTC580-BlockLib.');
      | disp(['Please check the parameters in the mask of ',gcb]);
      | disp('If you do not encounter any violations, then please ');
      | disp('copy the following lines and report this to support@ttcontrol.com ');
      | disp('<< begin of error message dump >>');
      | disp(['Version of TTC580-BlockLib: ', get_param(gcb,'tt_iolib_version')]);
      | disp(get_param(gcb,'ttDescription'));
      | disp(gcb);
      | x=lasterror;disp(x.message);
      | disp(get_param(gcb,'MaskValues'));
      | disp(version);
      | disp(computer);
      | disp('<< end of error message dump >>');
      | disp('------------------------------------------------------------');
      | disp(' ');
      | %Standard catch section END
      | end
      mask Callback bFlashOverEthernet:
      | try
      | s_ParameterDecision = 'bFlashOverEthernet'; %Deside on this parameter
      | c_ValuesDecision={'on'}; %Positive DescitionValues
      | s_ParameterInvisible = 'Enable_Reset_by_TTCDownloader'; %Make this invisible
      | %trim
      | if ischar(s_ParameterInvisible)%if secttion for compatibility reasons of template
      |     cs_ParameterInvisible = {s_ParameterInvisible};
      | else
      |     cs_ParameterInvisible = s_ParameterInvisible;
      | end
      | s_ParameterDecision = strtrim(s_ParameterDecision);
      | c_ValuesDecision = strtrim(c_ValuesDecision);
      | for j=1:length(cs_ParameterInvisible)
      |   s_ParameterInvisible = strtrim(cs_ParameterInvisible{j});
      |   c_MaskVisibilities=get_param(gcb,'MaskVisibilities');
      |   %check consistency
      |   idx=strmatch(s_ParameterInvisible,get_param(gcb,'MaskNames'),'exact');
      |   c_MaskVisibilities{idx}='on'; %default
      |     for i = 1: length(c_ValuesDecision)
      |         if ~isempty(strmatch(get_param(gcb, s_ParameterDecision), c_ValuesDecision{i},'exact'))
      |            c_MaskVisibilities{idx}='off';
      |         end
      |     end
      |   set_param(gcb,'MaskVisibilities',c_MaskVisibilities);
      | end
      | catch
      | %Standard catch section BEGIN
      | errordlg('An error occurred in a callback of the TTC580-BlockLib. Please open the Diagnostic Viewer for further details');
      | disp(' ');
      | disp('------------------------------------------------------------');
      | disp('An error occurred in a callback of the TTC580-BlockLib.');
      | disp(['Please check the parameters in the mask of ',gcb]);
      | disp('If you do not encounter any violations, then please ');
      | disp('copy the following lines and report this to support@ttcontrol.com ');
      | disp('<< begin of error message dump >>');
      | disp(['Version of TTC580-BlockLib: ', get_param(gcb,'tt_iolib_version')]);
      | disp(get_param(gcb,'ttDescription'));
      | disp(gcb);
      | x=lasterror;disp(x.message);
      | disp(get_param(gcb,'MaskValues'));
      | disp(version);
      | disp(computer);
      | disp('<< end of error message dump >>');
      | disp('------------------------------------------------------------');
      | disp(' ');
      | %Standard catch section END
      | end
      mask Callback Enable_CCP:
      | try
      | s_ParameterDecision = 'Enable_CCP'; %Deside on this parameter
      | c_ValuesDecision={'off'}; %Positive DescitionValues
      | s_ParameterInvisible = 'CRO_ID'; %Make this invisible
      | %trim
      | if ischar(s_ParameterInvisible)%if secttion for compatibility reasons of template
      |     cs_ParameterInvisible = {s_ParameterInvisible};
      | else
      |     cs_ParameterInvisible = s_ParameterInvisible;
      | end
      | s_ParameterDecision = strtrim(s_ParameterDecision);
      | c_ValuesDecision = strtrim(c_ValuesDecision);
      | for j=1:length(cs_ParameterInvisible)
      |   s_ParameterInvisible = strtrim(cs_ParameterInvisible{j});
      |   c_MaskVisibilities=get_param(gcb,'MaskVisibilities');
      |   %check consistency
      |   idx=strmatch(s_ParameterInvisible,get_param(gcb,'MaskNames'),'exact');
      |   c_MaskVisibilities{idx}='on'; %default
      |     for i = 1: length(c_ValuesDecision)
      |         if ~isempty(strmatch(get_param(gcb, s_ParameterDecision), c_ValuesDecision{i},'exact'))
      |            c_MaskVisibilities{idx}='off';
      |         end
      |     end
      |   set_param(gcb,'MaskVisibilities',c_MaskVisibilities);
      | end
      | s_ParameterDecision = 'Enable_CCP'; %Deside on this parameter
      | c_ValuesDecision={'off'}; %Positive DescitionValues
      | s_ParameterInvisible = 'DTO_ID'; %Make this invisible
      | %trim
      | if ischar(s_ParameterInvisible)%if secttion for compatibility reasons of template
      |     cs_ParameterInvisible = {s_ParameterInvisible};
      | else
      |     cs_ParameterInvisible = s_ParameterInvisible;
      | end
      | s_ParameterDecision = strtrim(s_ParameterDecision);
      | c_ValuesDecision = strtrim(c_ValuesDecision);
      | for j=1:length(cs_ParameterInvisible)
      |   s_ParameterInvisible = strtrim(cs_ParameterInvisible{j});
      |   c_MaskVisibilities=get_param(gcb,'MaskVisibilities');
      |   %check consistency
      |   idx=strmatch(s_ParameterInvisible,get_param(gcb,'MaskNames'),'exact');
      |   c_MaskVisibilities{idx}='on'; %default
      |     for i = 1: length(c_ValuesDecision)
      |         if ~isempty(strmatch(get_param(gcb, s_ParameterDecision), c_ValuesDecision{i},'exact'))
      |            c_MaskVisibilities{idx}='off';
      |         end
      |     end
      |   set_param(gcb,'MaskVisibilities',c_MaskVisibilities);
      | end
      | s_ParameterDecision = 'Enable_CCP'; %Deside on this parameter
      | c_ValuesDecision={'off'}; %Positive DescitionValues
      | s_ParameterInvisible = 'CCP_Station_Addr_raw'; %Make this invisible
      | %trim
      | if ischar(s_ParameterInvisible)%if secttion for compatibility reasons of template
      |     cs_ParameterInvisible = {s_ParameterInvisible};
      | else
      |     cs_ParameterInvisible = s_ParameterInvisible;
      | end
      | s_ParameterDecision = strtrim(s_ParameterDecision);
      | c_ValuesDecision = strtrim(c_ValuesDecision);
      | for j=1:length(cs_ParameterInvisible)
      |   s_ParameterInvisible = strtrim(cs_ParameterInvisible{j});
      |   c_MaskVisibilities=get_param(gcb,'MaskVisibilities');
      |   %check consistency
      |   idx=strmatch(s_ParameterInvisible,get_param(gcb,'MaskNames'),'exact');
      |   c_MaskVisibilities{idx}='on'; %default
      |     for i = 1: length(c_ValuesDecision)
      |         if ~isempty(strmatch(get_param(gcb, s_ParameterDecision), c_ValuesDecision{i},'exact'))
      |            c_MaskVisibilities{idx}='off';
      |         end
      |     end
      |   set_param(gcb,'MaskVisibilities',c_MaskVisibilities);
      | end
      | s_ParameterDecision = 'Enable_CCP'; %Deside on this parameter
      | c_ValuesDecision={'off'}; %Positive DescitionValues
      | s_ParameterInvisible = 'CCP_Station_ID'; %Make this invisible
      | %trim
      | if ischar(s_ParameterInvisible)%if secttion for compatibility reasons of template
      |     cs_ParameterInvisible = {s_ParameterInvisible};
      | else
      |     cs_ParameterInvisible = s_ParameterInvisible;
      | end
      | s_ParameterDecision = strtrim(s_ParameterDecision);
      | c_ValuesDecision = strtrim(c_ValuesDecision);
      | for j=1:length(cs_ParameterInvisible)
      |   s_ParameterInvisible = strtrim(cs_ParameterInvisible{j});
      |   c_MaskVisibilities=get_param(gcb,'MaskVisibilities');
      |   %check consistency
      |   idx=strmatch(s_ParameterInvisible,get_param(gcb,'MaskNames'),'exact');
      |   c_MaskVisibilities{idx}='on'; %default
      |     for i = 1: length(c_ValuesDecision)
      |         if ~isempty(strmatch(get_param(gcb, s_ParameterDecision), c_ValuesDecision{i},'exact'))
      |            c_MaskVisibilities{idx}='off';
      |         end
      |     end
      |   set_param(gcb,'MaskVisibilities',c_MaskVisibilities);
      | end
      | s_ParameterDecision = 'Enable_CCP'; %Deside on this parameter
      | c_ValuesDecision={'off'}; %Positive DescitionValues
      | s_ParameterInvisible = 'CPP_channel'; %Make this invisible
      | %trim
      | if ischar(s_ParameterInvisible)%if secttion for compatibility reasons of template
      |     cs_ParameterInvisible = {s_ParameterInvisible};
      | else
      |     cs_ParameterInvisible = s_ParameterInvisible;
      | end
      | s_ParameterDecision = strtrim(s_ParameterDecision);
      | c_ValuesDecision = strtrim(c_ValuesDecision);
      | for j=1:length(cs_ParameterInvisible)
      |   s_ParameterInvisible = strtrim(cs_ParameterInvisible{j});
      |   c_MaskVisibilities=get_param(gcb,'MaskVisibilities');
      |   %check consistency
      |   idx=strmatch(s_ParameterInvisible,get_param(gcb,'MaskNames'),'exact');
      |   c_MaskVisibilities{idx}='on'; %default
      |     for i = 1: length(c_ValuesDecision)
      |         if ~isempty(strmatch(get_param(gcb, s_ParameterDecision), c_ValuesDecision{i},'exact'))
      |            c_MaskVisibilities{idx}='off';
      |         end
      |     end
      |   set_param(gcb,'MaskVisibilities',c_MaskVisibilities);
      | end
      | s_ParameterDecision = 'Enable_CCP'; %Deside on this parameter
      | c_ValuesDecision={'off'}; %Positive DescitionValues
      | s_ParameterInvisible = 'CPP_id_format'; %Make this invisible
      | %trim
      | if ischar(s_ParameterInvisible)%if secttion for compatibility reasons of template
      |     cs_ParameterInvisible = {s_ParameterInvisible};
      | else
      |     cs_ParameterInvisible = s_ParameterInvisible;
      | end
      | s_ParameterDecision = strtrim(s_ParameterDecision);
      | c_ValuesDecision = strtrim(c_ValuesDecision);
      | for j=1:length(cs_ParameterInvisible)
      |   s_ParameterInvisible = strtrim(cs_ParameterInvisible{j});
      |   c_MaskVisibilities=get_param(gcb,'MaskVisibilities');
      |   %check consistency
      |   idx=strmatch(s_ParameterInvisible,get_param(gcb,'MaskNames'),'exact');
      |   c_MaskVisibilities{idx}='on'; %default
      |     for i = 1: length(c_ValuesDecision)
      |         if ~isempty(strmatch(get_param(gcb, s_ParameterDecision), c_ValuesDecision{i},'exact'))
      |            c_MaskVisibilities{idx}='off';
      |         end
      |     end
      |   set_param(gcb,'MaskVisibilities',c_MaskVisibilities);
      | end
      | s_ParameterDecision = 'Enable_CCP'; %Deside on this parameter
      | c_ValuesDecision={'off'}; %Positive DescitionValues
      | s_ParameterInvisible = 'bEnable_DAQ0'; %Make this invisible
      | %trim
      | if ischar(s_ParameterInvisible)%if secttion for compatibility reasons of template
      |     cs_ParameterInvisible = {s_ParameterInvisible};
      | else
      |     cs_ParameterInvisible = s_ParameterInvisible;
      | end
      | s_ParameterDecision = strtrim(s_ParameterDecision);
      | c_ValuesDecision = strtrim(c_ValuesDecision);
      | for j=1:length(cs_ParameterInvisible)
      |   s_ParameterInvisible = strtrim(cs_ParameterInvisible{j});
      |   c_MaskVisibilities=get_param(gcb,'MaskVisibilities');
      |   %check consistency
      |   idx=strmatch(s_ParameterInvisible,get_param(gcb,'MaskNames'),'exact');
      |   c_MaskVisibilities{idx}='on'; %default
      |     for i = 1: length(c_ValuesDecision)
      |         if ~isempty(strmatch(get_param(gcb, s_ParameterDecision), c_ValuesDecision{i},'exact'))
      |            c_MaskVisibilities{idx}='off';
      |         end
      |     end
      |   set_param(gcb,'MaskVisibilities',c_MaskVisibilities);
      | end
      | s_ParameterDecision = 'Enable_CCP'; %Deside on this parameter
      | c_ValuesDecision={'off'}; %Positive DescitionValues
      | s_ParameterInvisible = 'bEnable_DAQ1_2'; %Make this invisible
      | %trim
      | if ischar(s_ParameterInvisible)%if secttion for compatibility reasons of template
      |     cs_ParameterInvisible = {s_ParameterInvisible};
      | else
      |     cs_ParameterInvisible = s_ParameterInvisible;
      | end
      | s_ParameterDecision = strtrim(s_ParameterDecision);
      | c_ValuesDecision = strtrim(c_ValuesDecision);
      | for j=1:length(cs_ParameterInvisible)
      |   s_ParameterInvisible = strtrim(cs_ParameterInvisible{j});
      |   c_MaskVisibilities=get_param(gcb,'MaskVisibilities');
      |   %check consistency
      |   idx=strmatch(s_ParameterInvisible,get_param(gcb,'MaskNames'),'exact');
      |   c_MaskVisibilities{idx}='on'; %default
      |     for i = 1: length(c_ValuesDecision)
      |         if ~isempty(strmatch(get_param(gcb, s_ParameterDecision), c_ValuesDecision{i},'exact'))
      |            c_MaskVisibilities{idx}='off';
      |         end
      |     end
      |   set_param(gcb,'MaskVisibilities',c_MaskVisibilities);
      | end
      | s_ParameterDecision = 'Enable_CCP'; %Deside on this parameter
      | c_ValuesDecision={'off'}; %Positive DescitionValues
      | s_ParameterInvisible = 'ODT_total'; %Make this invisible
      | %trim
      | if ischar(s_ParameterInvisible)%if secttion for compatibility reasons of template
      |     cs_ParameterInvisible = {s_ParameterInvisible};
      | else
      |     cs_ParameterInvisible = s_ParameterInvisible;
      | end
      | s_ParameterDecision = strtrim(s_ParameterDecision);
      | c_ValuesDecision = strtrim(c_ValuesDecision);
      | for j=1:length(cs_ParameterInvisible)
      |   s_ParameterInvisible = strtrim(cs_ParameterInvisible{j});
      |   c_MaskVisibilities=get_param(gcb,'MaskVisibilities');
      |   %check consistency
      |   idx=strmatch(s_ParameterInvisible,get_param(gcb,'MaskNames'),'exact');
      |   c_MaskVisibilities{idx}='on'; %default
      |     for i = 1: length(c_ValuesDecision)
      |         if ~isempty(strmatch(get_param(gcb, s_ParameterDecision), c_ValuesDecision{i},'exact'))
      |            c_MaskVisibilities{idx}='off';
      |         end
      |     end
      |   set_param(gcb,'MaskVisibilities',c_MaskVisibilities);
      | end
      | s_ParameterDecision = 'Enable_CCP'; %Deside on this parameter
      | c_ValuesDecision={'on'}; %Positive DescitionValues
      | s_ParameterCB = 'bEnable_DAQ0'; %Run Callback of this parameter
      | %trim
      | if ischar(s_ParameterCB)%if secttion for compatibility reasons of template
      |     cs_ParameterCB = {s_ParameterCB};
      | else
      |     cs_ParameterCB = s_ParameterCB;
      | end
      | s_ParameterDecision = strtrim(s_ParameterDecision);
      | c_ValuesDecision = strtrim(c_ValuesDecision);
      | for j=1:length(cs_ParameterCB)
      |   s_ParameterCB = strtrim(cs_ParameterCB{j});
      |   c_MaskCallbacks=get_param(gcb,'MaskCallbacks');
      |   %check consistency
      |   idx=strmatch(s_ParameterCB,get_param(gcb,'MaskNames'),'exact');
      | %  c_MaskCallbacks{idx}='on'; %default
      |     for i = 1: length(c_ValuesDecision)
      |         if ~isempty(strmatch(get_param(gcb, s_ParameterDecision), c_ValuesDecision{i},'exact'))
      |            eval(c_MaskCallbacks{idx});
      |         end
      |     end
      | %  set_param(gcb,'MaskVisibilities',c_MaskCallbacks);
      | end
      | catch
      | %Standard catch section BEGIN
      | errordlg('An error occurred in a callback of the TTC580-BlockLib. Please open the Diagnostic Viewer for further details');
      | disp(' ');
      | disp('------------------------------------------------------------');
      | disp('An error occurred in a callback of the TTC580-BlockLib.');
      | disp(['Please check the parameters in the mask of ',gcb]);
      | disp('If you do not encounter any violations, then please ');
      | disp('copy the following lines and report this to support@ttcontrol.com ');
      | disp('<< begin of error message dump >>');
      | disp(['Version of TTC580-BlockLib: ', get_param(gcb,'tt_iolib_version')]);
      | disp(get_param(gcb,'ttDescription'));
      | disp(gcb);
      | x=lasterror;disp(x.message);
      | disp(get_param(gcb,'MaskValues'));
      | disp(version);
      | disp(computer);
      | disp('<< end of error message dump >>');
      | disp('------------------------------------------------------------');
      | disp(' ');
      | %Standard catch section END
      | end
      mask Callback CRO_ID:
      | try
      | %Check if given within bounds
      | if str2num(get_param(gcb,'CRO_ID')) > hex2dec('7FF')
      | error('CRO_ID Station ID needs to fit into a 11bit value (0x7FF) ')
      | end
      | catch
      | %Standard catch section BEGIN
      | errordlg('An error occurred in a callback of the TTC580-BlockLib. Please open the Diagnostic Viewer for further details');
      | disp(' ');
      | disp('------------------------------------------------------------');
      | disp('An error occurred in a callback of the TTC580-BlockLib.');
      | disp(['Please check the parameters in the mask of ',gcb]);
      | disp('If you do not encounter any violations, then please ');
      | disp('copy the following lines and report this to support@ttcontrol.com ');
      | disp('<< begin of error message dump >>');
      | disp(['Version of TTC580-BlockLib: ', get_param(gcb,'tt_iolib_version')]);
      | disp(get_param(gcb,'ttDescription'));
      | disp(gcb);
      | x=lasterror;disp(x.message);
      | disp(get_param(gcb,'MaskValues'));
      | disp(version);
      | disp(computer);
      | disp('<< end of error message dump >>');
      | disp('------------------------------------------------------------');
      | disp(' ');
      | %Standard catch section END
      | end
      mask Callback DTO_ID:
      | try
      | %Check if given within bounds
      | if str2num(get_param(gcb,'DTO_ID')) > hex2dec('7FF')
      | error('DTO_ID Station ID needs to fit into a 11bit value (0x7FF) ')
      | end
      | catch
      | %Standard catch section BEGIN
      | errordlg('An error occurred in a callback of the TTC580-BlockLib. Please open the Diagnostic Viewer for further details');
      | disp(' ');
      | disp('------------------------------------------------------------');
      | disp('An error occurred in a callback of the TTC580-BlockLib.');
      | disp(['Please check the parameters in the mask of ',gcb]);
      | disp('If you do not encounter any violations, then please ');
      | disp('copy the following lines and report this to support@ttcontrol.com ');
      | disp('<< begin of error message dump >>');
      | disp(['Version of TTC580-BlockLib: ', get_param(gcb,'tt_iolib_version')]);
      | disp(get_param(gcb,'ttDescription'));
      | disp(gcb);
      | x=lasterror;disp(x.message);
      | disp(get_param(gcb,'MaskValues'));
      | disp(version);
      | disp(computer);
      | disp('<< end of error message dump >>');
      | disp('------------------------------------------------------------');
      | disp(' ');
      | %Standard catch section END
      | end
      mask Callback CCP_Station_Addr_raw:
      | try
      | %Check if given within bounds
      | CCP_Station_Addr_raw_loc = str2num(get_param(gcb,'CCP_Station_Addr_raw'));
      | if or((CCP_Station_Addr_raw_loc> intmax('uint16')) , (CCP_Station_Addr_raw_loc < intmin('uint16')) )
      | error('CCP Station ID needs to fit into a uint16 value')
      | %possible clash with data dictionary moved from Callback to MaskInitialisation
      | %CCP_Station_Addr = 0; % some value
      | %else
      | %CCP_Station_Addr = swapbytes(uint16(CCP_Station_Addr_raw_loc));%because of big-endian format on the TMS570
      | end
      | catch
      | %Standard catch section BEGIN
      | errordlg('An error occurred in a callback of the TTC580-BlockLib. Please open the Diagnostic Viewer for further details');
      | disp(' ');
      | disp('------------------------------------------------------------');
      | disp('An error occurred in a callback of the TTC580-BlockLib.');
      | disp(['Please check the parameters in the mask of ',gcb]);
      | disp('If you do not encounter any violations, then please ');
      | disp('copy the following lines and report this to support@ttcontrol.com ');
      | disp('<< begin of error message dump >>');
      | disp(['Version of TTC580-BlockLib: ', get_param(gcb,'tt_iolib_version')]);
      | disp(get_param(gcb,'ttDescription'));
      | disp(gcb);
      | x=lasterror;disp(x.message);
      | disp(get_param(gcb,'MaskValues'));
      | disp(version);
      | disp(computer);
      | disp('<< end of error message dump >>');
      | disp('------------------------------------------------------------');
      | disp(' ');
      | %Standard catch section END
      | end
      mask Callback CCP_Station_ID: %
      mask TypeOptions CPP_channel: IO_CAN_CHANNEL_0  | IO_CAN_CHANNEL_1 | IO_CAN_CHANNEL_2
      mask Callback CPP_channel: %
      mask TypeOptions CPP_id_format: IO_CAN_STD_FRAME | IO_CAN_EXT_FRAME
      mask Callback CPP_id_format: %
      mask Callback bEnable_DAQ0:
      | try
      | s_ParameterDecision = {'bEnable_DAQ0','bEnable_DAQ1_2'}; %Deside on this parameter
      | c_ValuesDecision={'off'}; %Positive DescitionValues
      | s_ParameterInvisible = 'ODT_total'; %Make this invisible
      | %trim
      | if ischar(s_ParameterInvisible)%if secttion for compatibility reasons of template
      |     cs_ParameterInvisible = {s_ParameterInvisible};
      | else
      |     cs_ParameterInvisible = s_ParameterInvisible;
      | end
      | if ischar(s_ParameterDecision)%if secttion for compatibility reasons of template
      |     cs_ParameterDecision = {s_ParameterDecision};
      | else
      |     cs_ParameterDecision = s_ParameterDecision;
      | end
      | cs_ParameterDecision = strtrim(cs_ParameterDecision);
      | c_ValuesDecision = strtrim(c_ValuesDecision);
      | for j=1:length(cs_ParameterInvisible)
      |     s_ParameterInvisible = strtrim(cs_ParameterInvisible{j});
      |     c_MaskVisibilities=get_param(gcb,'MaskVisibilities');
      |     %check consistency
      |     idx=strmatch(s_ParameterInvisible,get_param(gcb,'MaskNames'),'exact');
      |     if (length(cs_ParameterDecision) == 1)  %single decision value: original
      |         c_MaskVisibilities{idx}='on'; %default
      |         for i = 1: length(c_ValuesDecision)
      |             if ~isempty(strmatch(get_param(gcb, cs_ParameterDecision{1}), c_ValuesDecision{i},'exact'))
      |                 c_MaskVisibilities{idx}='off';
      |             end
      |         end
      |     else
      |         c_MaskVisibilities{idx}='off';  %multiple decision: new default
      |         for i = 1: length(cs_ParameterDecision)
      |             if ~any(strcmp(get_param(gcb, cs_ParameterDecision{i}), c_ValuesDecision))
      |                 c_MaskVisibilities{idx}='on';
      |             end
      |         end
      |     end
      |     set_param(gcb,'MaskVisibilities',c_MaskVisibilities);
      | end
      | 
      | catch
      | %Standard catch section BEGIN
      | errordlg('An error occurred in a callback of the TTC580-BlockLib. Please open the Diagnostic Viewer for further details');
      | disp(' ');
      | disp('------------------------------------------------------------');
      | disp('An error occurred in a callback of the TTC580-BlockLib.');
      | disp(['Please check the parameters in the mask of ',gcb]);
      | disp('If you do not encounter any violations, then please ');
      | disp('copy the following lines and report this to support@ttcontrol.com ');
      | disp('<< begin of error message dump >>');
      | disp(['Version of TTC580-BlockLib: ', get_param(gcb,'tt_iolib_version')]);
      | disp(get_param(gcb,'ttDescription'));
      | disp(gcb);
      | x=lasterror;disp(x.message);
      | disp(get_param(gcb,'MaskValues'));
      | disp(version);
      | disp(computer);
      | disp('<< end of error message dump >>');
      | disp('------------------------------------------------------------');
      | disp(' ');
      | %Standard catch section END
      | end
      mask Callback bEnable_DAQ1_2:
      | try
      | s_ParameterDecision = {'bEnable_DAQ0','bEnable_DAQ1_2'}; %Deside on this parameter
      | c_ValuesDecision={'off'}; %Positive DescitionValues
      | s_ParameterInvisible = 'ODT_total'; %Make this invisible
      | %trim
      | if ischar(s_ParameterInvisible)%if secttion for compatibility reasons of template
      |     cs_ParameterInvisible = {s_ParameterInvisible};
      | else
      |     cs_ParameterInvisible = s_ParameterInvisible;
      | end
      | if ischar(s_ParameterDecision)%if secttion for compatibility reasons of template
      |     cs_ParameterDecision = {s_ParameterDecision};
      | else
      |     cs_ParameterDecision = s_ParameterDecision;
      | end
      | cs_ParameterDecision = strtrim(cs_ParameterDecision);
      | c_ValuesDecision = strtrim(c_ValuesDecision);
      | for j=1:length(cs_ParameterInvisible)
      |     s_ParameterInvisible = strtrim(cs_ParameterInvisible{j});
      |     c_MaskVisibilities=get_param(gcb,'MaskVisibilities');
      |     %check consistency
      |     idx=strmatch(s_ParameterInvisible,get_param(gcb,'MaskNames'),'exact');
      |     if (length(cs_ParameterDecision) == 1)  %single decision value: original
      |         c_MaskVisibilities{idx}='on'; %default
      |         for i = 1: length(c_ValuesDecision)
      |             if ~isempty(strmatch(get_param(gcb, cs_ParameterDecision{1}), c_ValuesDecision{i},'exact'))
      |                 c_MaskVisibilities{idx}='off';
      |             end
      |         end
      |     else
      |         c_MaskVisibilities{idx}='off';  %multiple decision: new default
      |         for i = 1: length(cs_ParameterDecision)
      |             if ~any(strcmp(get_param(gcb, cs_ParameterDecision{i}), c_ValuesDecision))
      |                 c_MaskVisibilities{idx}='on';
      |             end
      |         end
      |     end
      |     set_param(gcb,'MaskVisibilities',c_MaskVisibilities);
      | end
      | 
      | catch
      | %Standard catch section BEGIN
      | errordlg('An error occurred in a callback of the TTC580-BlockLib. Please open the Diagnostic Viewer for further details');
      | disp(' ');
      | disp('------------------------------------------------------------');
      | disp('An error occurred in a callback of the TTC580-BlockLib.');
      | disp(['Please check the parameters in the mask of ',gcb]);
      | disp('If you do not encounter any violations, then please ');
      | disp('copy the following lines and report this to support@ttcontrol.com ');
      | disp('<< begin of error message dump >>');
      | disp(['Version of TTC580-BlockLib: ', get_param(gcb,'tt_iolib_version')]);
      | disp(get_param(gcb,'ttDescription'));
      | disp(gcb);
      | x=lasterror;disp(x.message);
      | disp(get_param(gcb,'MaskValues'));
      | disp(version);
      | disp(computer);
      | disp('<< end of error message dump >>');
      | disp('------------------------------------------------------------');
      | disp(' ');
      | %Standard catch section END
      | end
      mask Callback ODT_total:
      | try
      | sParam = 'ODT_total';
      | vBounds = [1,254];
      | Param = get_param(gcb,sParam);
      | if isstr(Param)
      |     iValue = str2num(Param);
      | elseif isnumeric(Param)
      |     iValue = Param;
      | else
      |    error(['Type of ',sParam,' is wrong!']);
      | end
      | if or( (any(iValue < vBounds(1))) , (any(iValue > vBounds(2))) )
      |     error(['Value of ',sParam,' is chosen out of bounds [',num2str(vBounds(1)),'..',num2str(vBounds(2)),']']);
      | end
      | catch
      | %Standard catch section BEGIN
      | errordlg('An error occurred in a callback of the TTC580-BlockLib. Please open the Diagnostic Viewer for further details');
      | disp(' ');
      | disp('------------------------------------------------------------');
      | disp('An error occurred in a callback of the TTC580-BlockLib.');
      | disp(['Please check the parameters in the mask of ',gcb]);
      | disp('If you do not encounter any violations, then please ');
      | disp('copy the following lines and report this to support@ttcontrol.com ');
      | disp('<< begin of error message dump >>');
      | disp(['Version of TTC580-BlockLib: ', get_param(gcb,'tt_iolib_version')]);
      | disp(get_param(gcb,'ttDescription'));
      | disp(gcb);
      | x=lasterror;disp(x.message);
      | disp(get_param(gcb,'MaskValues'));
      | disp(version);
      | disp(computer);
      | disp('<< end of error message dump >>');
      | disp('------------------------------------------------------------');
      | disp(' ');
      | %Standard catch section END
      | end
      mask Callback bEnable_ErrorCBAction:
      | try
      | s_ParameterDecision = 'bEnable_ErrorCBAction'; %Deside on this parameter
      | c_ValuesDecision={'off'}; %Positive DescitionValues
      | s_ParameterInvisible = 'bDIAG_ERR_DISABLE_SSW0'; %Make this invisible
      | %trim
      | if ischar(s_ParameterInvisible)%if secttion for compatibility reasons of template
      |     cs_ParameterInvisible = {s_ParameterInvisible};
      | else
      |     cs_ParameterInvisible = s_ParameterInvisible;
      | end
      | s_ParameterDecision = strtrim(s_ParameterDecision);
      | c_ValuesDecision = strtrim(c_ValuesDecision);
      | for j=1:length(cs_ParameterInvisible)
      |   s_ParameterInvisible = strtrim(cs_ParameterInvisible{j});
      |   c_MaskVisibilities=get_param(gcb,'MaskVisibilities');
      |   %check consistency
      |   idx=strmatch(s_ParameterInvisible,get_param(gcb,'MaskNames'),'exact');
      |   c_MaskVisibilities{idx}='on'; %default
      |     for i = 1: length(c_ValuesDecision)
      |         if ~isempty(strmatch(get_param(gcb, s_ParameterDecision), c_ValuesDecision{i},'exact'))
      |            c_MaskVisibilities{idx}='off';
      |         end
      |     end
      |   set_param(gcb,'MaskVisibilities',c_MaskVisibilities);
      | end
      | s_ParameterDecision = 'bEnable_ErrorCBAction'; %Deside on this parameter
      | c_ValuesDecision={'off'}; %Positive DescitionValues
      | s_ParameterInvisible = 'bDIAG_ERR_DISABLE_SSW1'; %Make this invisible
      | %trim
      | if ischar(s_ParameterInvisible)%if secttion for compatibility reasons of template
      |     cs_ParameterInvisible = {s_ParameterInvisible};
      | else
      |     cs_ParameterInvisible = s_ParameterInvisible;
      | end
      | s_ParameterDecision = strtrim(s_ParameterDecision);
      | c_ValuesDecision = strtrim(c_ValuesDecision);
      | for j=1:length(cs_ParameterInvisible)
      |   s_ParameterInvisible = strtrim(cs_ParameterInvisible{j});
      |   c_MaskVisibilities=get_param(gcb,'MaskVisibilities');
      |   %check consistency
      |   idx=strmatch(s_ParameterInvisible,get_param(gcb,'MaskNames'),'exact');
      |   c_MaskVisibilities{idx}='on'; %default
      |     for i = 1: length(c_ValuesDecision)
      |         if ~isempty(strmatch(get_param(gcb, s_ParameterDecision), c_ValuesDecision{i},'exact'))
      |            c_MaskVisibilities{idx}='off';
      |         end
      |     end
      |   set_param(gcb,'MaskVisibilities',c_MaskVisibilities);
      | end
      | s_ParameterDecision = 'bEnable_ErrorCBAction'; %Deside on this parameter
      | c_ValuesDecision={'off'}; %Positive DescitionValues
      | s_ParameterInvisible = 'bDIAG_ERR_DISABLE_SSW2'; %Make this invisible
      | %trim
      | if ischar(s_ParameterInvisible)%if secttion for compatibility reasons of template
      |     cs_ParameterInvisible = {s_ParameterInvisible};
      | else
      |     cs_ParameterInvisible = s_ParameterInvisible;
      | end
      | s_ParameterDecision = strtrim(s_ParameterDecision);
      | c_ValuesDecision = strtrim(c_ValuesDecision);
      | for j=1:length(cs_ParameterInvisible)
      |   s_ParameterInvisible = strtrim(cs_ParameterInvisible{j});
      |   c_MaskVisibilities=get_param(gcb,'MaskVisibilities');
      |   %check consistency
      |   idx=strmatch(s_ParameterInvisible,get_param(gcb,'MaskNames'),'exact');
      |   c_MaskVisibilities{idx}='on'; %default
      |     for i = 1: length(c_ValuesDecision)
      |         if ~isempty(strmatch(get_param(gcb, s_ParameterDecision), c_ValuesDecision{i},'exact'))
      |            c_MaskVisibilities{idx}='off';
      |         end
      |     end
      |   set_param(gcb,'MaskVisibilities',c_MaskVisibilities);
      | end
      | catch
      | %Standard catch section BEGIN
      | errordlg('An error occurred in a callback of the TTC580-BlockLib. Please open the Diagnostic Viewer for further details');
      | disp(' ');
      | disp('------------------------------------------------------------');
      | disp('An error occurred in a callback of the TTC580-BlockLib.');
      | disp(['Please check the parameters in the mask of ',gcb]);
      | disp('If you do not encounter any violations, then please ');
      | disp('copy the following lines and report this to support@ttcontrol.com ');
      | disp('<< begin of error message dump >>');
      | disp(['Version of TTC580-BlockLib: ', get_param(gcb,'tt_iolib_version')]);
      | disp(get_param(gcb,'ttDescription'));
      | disp(gcb);
      | x=lasterror;disp(x.message);
      | disp(get_param(gcb,'MaskValues'));
      | disp(version);
      | disp(computer);
      | disp('<< end of error message dump >>');
      | disp('------------------------------------------------------------');
      | disp(' ');
      | %Standard catch section END
      | end
      mask Callback bDIAG_ERR_DISABLE_SSW0: %
      mask Callback bDIAG_ERR_DISABLE_SSW1: %
      mask Callback bDIAG_ERR_DISABLE_SSW2: %
  Postrun_Enable : Subsystem  LoadFcn=|  mask(Postrun_Enable_Code){SampleTime=-1, ttlib=IO_Blk_Lib_TTC500, ttDescription=Postrun_Enable, tt_iolib_version=0.26}
      | try
      | %
      | %Upgrade Information - standard BEGIN
      | new_color = 'blue';
      | new_ver = '0.26';
      | act_ver = get_param(gcb,'tt_iolib_version');
      | if not(strcmp(act_ver,new_ver))
      |     disp(['Upgrade block: ',gcb,char(10),'       Version: ',act_ver,' to ',new_ver]);
      |     %switch - case for specific upgrade information e.g. additional parameter required 
      |     %Change appearance and version information
      |     set_param(gcb,'ForegroundColor',new_color);
      |     set_param(gcb,'tt_iolib_version',new_ver);
      | end
      | %Upgrade Information - standard END
      | catch
      | %Standard catch section BEGIN
      | errordlg('An error occurred in a callback of the TTC580-BlockLib. Please open the Diagnostic Viewer for further details');
      | disp(' ');
      | disp('------------------------------------------------------------');
      | disp('An error occurred in a callback of the TTC580-BlockLib.');
      | disp(['Please check the parameters in the mask of ',gcb]);
      | disp('If you do not encounter any violations, then please '); 
      | disp('copy the following lines and report this to support@ttcontrol.com ');
      | disp('<< begin of error message dump >>');
      | disp(['Version of TTC580-BlockLib: ', get_param(gcb,'tt_iolib_version')]);
      | disp(get_param(gcb,'ttDescription'));
      | disp(gcb);
      | x=lasterror;disp(x.message);
      | disp(get_param(gcb,'MaskValues'));
      | disp(version);
      | disp(computer);
      | disp('<< end of error message dump >>');
      | disp('------------------------------------------------------------');
      | disp(' ');
      | %Standard catch section END
      | end
      mask help: Enables postrun of the ECU
      mask init: same as IOBlock_Library_TTC580/ADC Blocks TTC580 IOlib/ADC_Absolute_10V
      settings: CopyFcn=%deleted
      mask Help: web([which('usermanual.html'),'#',lower(get_param(gcb,'ttDescription'))])
  Power_Enable : Subsystem  LoadFcn=|  mask(Power_Enable_Code){SampleTime=-1, ttlib=IO_Blk_Lib_TTC500, ttDescription=Power_Enable, tt_iolib_version=0.26}
      | try
      | %
      | %Upgrade Information - standard BEGIN
      | new_color = 'blue';
      | new_ver = '0.26';
      | act_ver = get_param(gcb,'tt_iolib_version');
      | if not(strcmp(act_ver,new_ver))
      |     disp(['Upgrade block: ',gcb,char(10),'       Version: ',act_ver,' to ',new_ver]);
      |     %switch - case for specific upgrade information e.g. additional parameter required 
      |     %Change appearance and version information
      |     set_param(gcb,'ForegroundColor',new_color);
      |     set_param(gcb,'tt_iolib_version',new_ver);
      | end
      | %Upgrade Information - standard END
      | catch
      | %Standard catch section BEGIN
      | errordlg('An error occurred in a callback of the TTC580-BlockLib. Please open the Diagnostic Viewer for further details');
      | disp(' ');
      | disp('------------------------------------------------------------');
      | disp('An error occurred in a callback of the TTC580-BlockLib.');
      | disp(['Please check the parameters in the mask of ',gcb]);
      | disp('If you do not encounter any violations, then please '); 
      | disp('copy the following lines and report this to support@ttcontrol.com ');
      | disp('<< begin of error message dump >>');
      | disp(['Version of TTC580-BlockLib: ', get_param(gcb,'tt_iolib_version')]);
      | disp(get_param(gcb,'ttDescription'));
      | disp(gcb);
      | x=lasterror;disp(x.message);
      | disp(get_param(gcb,'MaskValues'));
      | disp(version);
      | disp(computer);
      | disp('<< end of error message dump >>');
      | disp('------------------------------------------------------------');
      | disp(' ');
      | %Standard catch section END
      | end
      mask help: Enables all power outputs
      mask init: same as IOBlock_Library_TTC580/ADC Blocks TTC580 IOlib/ADC_Absolute_10V
      settings: CopyFcn=%deleted
      mask Help: web([which('usermanual.html'),'#',lower(get_param(gcb,'ttDescription'))])
  SetDateAndTime : Subsystem  LoadFcn=|  mask(SetDateAndTime_Code){SampleTime=-1, ttlib=IO_Blk_Lib_TTC500, ttDescription=SetDateAndTime, tt_iolib_version=0.18}
      | try
      | %
      | %Upgrade Information - standard BEGIN
      | new_color = 'blue';
      | new_ver = '0.18';
      | act_ver = get_param(gcb,'tt_iolib_version');
      | if not(strcmp(act_ver,new_ver))
      |     disp(['Upgrade block: ',gcb,char(10),'       Version: ',act_ver,' -> ',new_ver]);
      |     %switch - case for specific upgrade information e.g. additional parameter required 
      |     %Change appearance and version information
      |     set_param(gcb,'ForegroundColor',new_color);
      |     set_param(gcb,'tt_iolib_version',new_ver);
      | end
      | %Upgrade Information - standard END
      | catch
      | %Standard catch section BEGIN 
      | disp(' ');
      | disp('------------------------------------------------------------');
      | disp('An error occurred in a callback of the TTC580-BlockLib.');
      | disp(['Please check the parameters in the mask of ',gcb]);
      | disp('If you do not encounter any violations, then please '); 
      | disp('copy the following lines and report this to support@ttcontrol.com ');
      | disp('<< begin of error message dump >>');
      | disp(['Version of TTC580-BlockLib: ', get_param(gcb,'tt_iolib_version')]);
      | disp(get_param(gcb,'ttDescription'));
      | disp(gcb);
      | x=lasterror;disp(x.message);
      | disp(get_param(gcb,'MaskValues'));
      | disp(version);
      | disp(computer);
      | disp('<< end of error message dump >>');
      | disp('------------------------------------------------------------');
      | disp(' ');
      | %Standard catch section END
      | end
      mask help: Sets the date and time of the real time clock.
      mask init:
      | %
      settings: CopyFcn=%deleted
      mask Help: web([which('usermanual.html'),'#',lower(get_param(gcb,'ttDescription'))])
  compare2error : Subsystem  LoadFcn=|  mask(compare2error_Code){SampleTime=-1, ttlib=IO_Blk_Lib_TTC500, ttDescription=compare2error, tt_iolib_version=0.19, define=IO_E_OK}
      | try
      | %
      | %Upgrade Information - standard BEGIN
      | new_color = 'blue';
      | new_ver = '0.19';
      | act_ver = get_param(gcb,'tt_iolib_version');
      | if not(strcmp(act_ver,new_ver))
      |     disp(['Upgrade block: ',gcb,char(10),'       Version: ',act_ver,' -> ',new_ver]);
      |     %switch - case for specific upgrade information e.g. additional parameter required 
      |     %Change appearance and version information
      |     set_param(gcb,'ForegroundColor',new_color);
      |     set_param(gcb,'tt_iolib_version',new_ver);
      | end
      | %Upgrade Information - standard END
      | catch
      | %Standard catch section BEGIN 
      | disp(' ');
      | disp('------------------------------------------------------------');
      | disp('An error occurred in a callback of the TTC580-BlockLib.');
      | disp(['Please check the parameters in the mask of ',gcb]);
      | disp('If you do not encounter any violations, then please '); 
      | disp('copy the following lines and report this to support@ttcontrol.com ');
      | disp('<< begin of error message dump >>');
      | disp(['Version of TTC580-BlockLib: ', get_param(gcb,'tt_iolib_version')]);
      | disp(get_param(gcb,'ttDescription'));
      | disp(gcb);
      | x=lasterror;disp(x.message);
      | disp(get_param(gcb,'MaskValues'));
      | disp(version);
      | disp(computer);
      | disp('<< end of error message dump >>');
      | disp('------------------------------------------------------------');
      | disp(' ');
      | %Standard catch section END
      | end
      mask help: Check of ErrorCode
      mask init:
      | %
      settings: CopyFcn=%deleted
      mask Help: web([which('usermanual.html'),'#',lower(get_param(gcb,'ttDescription'))])
      mask TypeOptions define: IO_E_OK | IO_E_BUSY | IO_E_UNKNOWN | IO_E_DRV_SAFETY_CONF_NOT_CONFIG | IO_E_INVALID_SAFETY_CONFIG | IO_E_DRV_SAFETY_CYCLE_RUNNING | IO_E_OPEN_LOAD | IO_E_SHORT_GND | IO_E_SHORT_BAT | IO_E_OPEN_LOAD_OR_SHORT_BAT | IO_E_INVALID_VOLTAGE | IO_E_PWM_NO_DIAG | IO_E_STARTUP | IO_E_SAFE_STATE | IO_E_REFERENCE | IO_E_SAFETY_SWITCH_DISABLED | IO_E_FET_PROT_ACTIVE | IO_E_FET_PROT_PERMANENT | IO_E_FET_PROT_REENABLE | IO_E_FET_PROT_WAIT | IO_E_FET_PROT_NOT_ACTIVE | IO_E_NULL_POINTER | IO_E_INVALID_PARAMETER | IO_E_CHANNEL_BUSY | IO_E_CHANNEL_NOT_CONFIGURED | IO_E_INVALID_CHANNEL_ID | IO_E_INVALID_LIMITS | IO_E_PERIODIC_NOT_CONFIGURED | IO_E_CH_CAPABILITY | IO_E_DRIVER_NOT_INITIALIZED | IO_E_CAN_OVERFLOW | IO_E_CAN_WRONG_HANDLE | IO_E_CAN_MAX_MO_REACHED | IO_E_CAN_MAX_HANDLES_REACHED | IO_E_CAN_FIFO_FULL | IO_E_CAN_OLD_DATA | IO_E_CAN_ERROR_PASSIVE | IO_E_CAN_BUS_OFF | IO_E_CAN_ERROR_WARNING | IO_E_CAN_TIMEOUT | IO_E_EEPROM_RANGE | IO_E_UART_BUFFER_FULL | IO_E_UART_BUFFER_EMPTY | IO_E_UART_OVERFLOW | IO_E_UART_PARITY | IO_E_UART_FRAMING | IO_E_PWD_NOT_FINISHED | IO_E_PWD_OVERFLOW | IO_E_PWD_CURRENT_THRESH_HIGH | IO_E_PWD_CURRENT_THRESH_LOW | IO_E_CM_CALIBRATION | IO_E_FPGA_NOT_INITIALIZED | IO_E_FPGA_TIMEOUT | IO_E_FPGA_CRC_ERROR | IO_E_FPGA_VERSION | IO_E_WD_RANGE | IO_E_WD_INITIALIZATION | IO_E_WD_PRECISION | IO_E_WD_ACTIVATION | IO_E_WD_TRIGGER | IO_E_WD_SAFE_LOCK | IO_E_WD_DEBUGGING_PREPARED | IO_E_WD_SELF_MONITORING | IO_E_WD_VICE_VERSA_MONITORING | IO_E_WD_STATUS_INVALID | IO_E_RTC_CLOCK_INTEGRITY_FAILED | IO_E_LIN_BIT | IO_E_LIN_PHYSICAL_BUS | IO_E_LIN_CHECKSUM | IO_E_LIN_INCONSISTENT_SYNCH_FIELD | IO_E_LIN_NO_RESPONSE | IO_E_LIN_FRAMING | IO_E_LIN_OVERRUN | IO_E_LIN_PARITY | IO_E_LIN_TIMEOUT | IO_E_FLASH_WRONG_DEVICE_ID | IO_E_FLASH_BLANK_CHECK_FAILED | IO_E_FLASH_OP_FAILED | IO_E_FLASH_OP_TIMEOUT | IO_E_INVALID_VARIANT | IO_E_INVALID_PROD_DATA | IO_E_INVALID_PIN_CONFIG | IO_E_INVALID_SERIAL_NUMBER | IO_E_CORE_TEST_FAILED | IO_E_ERROR_PIN_TEST_TIMEOUT | IO_E_ERROR_PIN_TEST_FAILED | IO_E_INTERNAL_MEM_FAILED | IO_E_INVALID_ESM_INIT_STATUS | IO_E_INTERNAL_CSM | IO_E_ETH_INIT_FAIL | IO_E_ETH_INIT_TIMEOUT | IO_E_ETH_DEINIT_TIMEOUT | IO_E_ETH_MAC_INVALID | IO_E_ETH_READ_FAIL | IO_E_ETH_WRITE_FAIL | IO_E_ETH_NO_LINK | IO_E_ETH_MDIO_TIMEOUT | IO_E_ETH_MDIO_READ | IO_E_DOWNLOAD_NO_REQ | IO_E_DOWNLOAD_TIMEOUT | IO_E_DOWNLOAD_HANDSHAKE | IO_E_SHM_INTEGRITY | IO_E_MPU_REGION_ENABLED | IO_E_MPU_REGION_DISABLED
      mask Callback define: %
